simulink model "StopwatchAra2016"  (R2017b)
settings: Solver=ode3  StartTime=0.0  StopTime=Inf  RelTol=1e-3
libraries: simulink x1
settings Model: Creator=Gabriele Ara  LastModifiedBy=gabriele
settings OptimizationCC: DefaultParameterBehavior=Inlined  InlineInvariantSignals=on
settings DebuggingCC: ParameterTunabilityLossMsg=error
settings SFSimCC: MATLABDynamicMemAlloc=off
settings RTWCC: SystemTargetFile=ert.tlc  GenCodeOnly=on  TemplateMakefile=ert_default_tmf  GenerateReport=on  IncludeHyperlinkInReport=on  LaunchReport=on  GenerateTraceInfo=on  GenerateTraceReport=on  GenerateTraceReportSl=on  GenerateTraceReportSf=on  GenerateTraceReportEml=on
settings CodeAppCC: ForceParamTrailComments=on  IgnoreCustomStorageClasses=off  OperatorAnnotations=on  SimulinkDataObjDesc=on  SFDataObjDesc=on  MATLABFcnDesc=on  InsertBlockDesc=on  StateflowObjectComments=on  MATLABSourceComments=on
settings ERTTargetCC: TargetLangStandard=C99 (ISO)  MultiwordLength=2048  GenerateSampleERTMain=on  SupportAbsoluteTime=off  MultiInstanceERTCode=on  CodeInterfacePackaging=Reusable function  SupportNonFinite=off  SupportComplex=off  PurelyIntegerCode=on  InlinedParameterPlacement=NonHierarchical  MultiInstanceErrorCode=None  ERTCustomFileTemplate=example_file_process.tlc

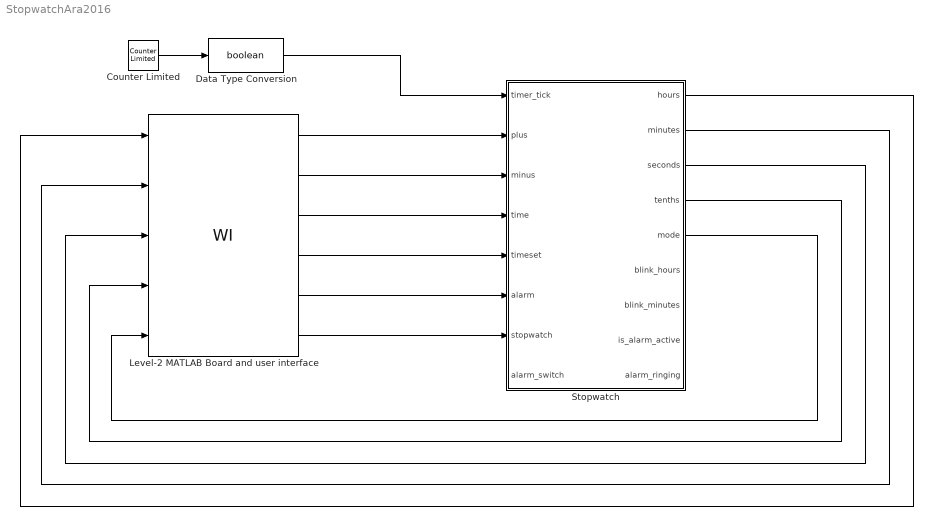
== system StopwatchAra2016 ==
  Counter Limited : simulink/Sources/Counter Limited  uplimit=1  tsamp=0.1
  Data Type Conversion : DataTypeConversion  OutDataTypeStr=boolean
  Level-2 MATLAB Board and user interface : M-S-Function  FunctionName=WI
      mask Display:
      | port_label('input', 1, 'hours')
      | port_label('input', 2, 'minutes')
      | port_label('input', 3, 'seconds')
      | port_label('input', 4, 'tenths')
      | port_label('input', 5, 'mode')
      | 
      | port_label('output', 1, 'plus')
      | port_label('output', 2, 'minus')
      | port_label('output', 3, 'time')
      | port_label('output', 4, 'time_set')
      | port_label('output', 5, 'alarm')
      | port_label('output', 6, 'stopwatch')
  Stopwatch : Subsystem
  wires:
  Level-2 MATLAB Board and user interface/1 -> Stopwatch/2(plus)
  Level-2 MATLAB Board and user interface/2 -> Stopwatch/3(minus)
  Level-2 MATLAB Board and user interface/3 -> Stopwatch/4(time)
  Level-2 MATLAB Board and user interface/4 -> Stopwatch/5(timeset)
  Level-2 MATLAB Board and user interface/5 -> Stopwatch/6(alarm)
  Level-2 MATLAB Board and user interface/6 -> Stopwatch/7(stopwatch)
  Stopwatch/1(hours) -> Level-2 MATLAB Board and user interface/1
  Stopwatch/2(minutes) -> Level-2 MATLAB Board and user interface/2
  Stopwatch/3(seconds) -> Level-2 MATLAB Board and user interface/3
  Stopwatch/4(tenths) -> Level-2 MATLAB Board and user interface/4
  Stopwatch/5(mode) -> Level-2 MATLAB Board and user interface/5
  Data Type Conversion/1 -> Stopwatch/1(timer_tick)
  Counter Limited/1 -> Data Type Conversion/1

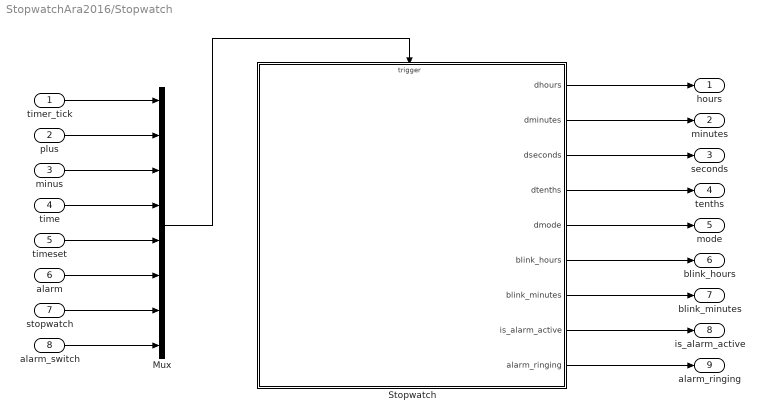
== system StopwatchAra2016/Stopwatch ==
  timer_tick : Inport
  plus : Inport  Port=2
  minus : Inport  Port=3
  time : Inport  Port=4
  timeset : Inport  Port=5
  alarm : Inport  Port=6
  stopwatch : Inport  Port=7
  alarm_switch : Inport  Port=8
  Mux : Mux  Inputs=8
  Stopwatch : Stateflow chart  TreatAsAtomicUnit=on
  hours : Outport
  minutes : Outport  Port=2
  seconds : Outport  Port=3
  tenths : Outport  Port=4
  mode : Outport  Port=5
  blink_hours : Outport  Port=6
  blink_minutes : Outport  Port=7
  is_alarm_active : Outport  Port=8
  alarm_ringing : Outport  Port=9
  wires:
  plus/1 -> Mux/2
  Stopwatch/1(dhours) -> hours/1
  minus/1 -> Mux/3
  timeset/1 -> Mux/5
  alarm/1 -> Mux/6
  time/1 -> Mux/4
  stopwatch/1 -> Mux/7
  Stopwatch/2(dminutes) -> minutes/1
  Stopwatch/5(dmode) -> mode/1
  Stopwatch/4(dtenths) -> tenths/1
  Stopwatch/3(dseconds) -> seconds/1
  Mux/1 -> Stopwatch/Trigger
  Stopwatch/8(is_alarm_active) -> is_alarm_active/1
  Stopwatch/7(blink_minutes) -> blink_minutes/1
  Stopwatch/6(blink_hours) -> blink_hours/1
  Stopwatch/9(alarm_ringing) -> alarm_ringing/1
  alarm_switch/1 -> Mux/8
  timer_tick/1 -> Mux/1

== stateflow chart StopwatchAra2016/Stopwatch/Stopwatch ==
  settings: executeAtInitialization=1
  state Control [parallel]
    en: blink_hours = uint8(0); blink_minutes = uint8(0);
    settings: executionOrder=1
    state timemode
      en: dmode = uint8(0);
      du: dhours = hours; dminutes = minutes; dseconds = seconds; dtenths = tenths;
    state timesetmode
      en: dmode = uint8(1); dhours = hours; dminutes = minutes;
      ex: hours = dhours; minutes = dminutes;
      state setMinutes
        en: blink_minutes = uint8(1);
        ex: blink_minutes = uint8(0);
        setMinutes -> setMinutes [order 1] : bplus {dminutes = mod(dminutes + 1, 60)}
        setMinutes -> setMinutes [order 2] : bminus [dminutes == 0]{dminutes = uint8(59)}
        setMinutes -> setMinutes [order 3] : bminus {dminutes = dminutes - 1}
      state setHours
        en: blink_hours = uint8(1);
        ex: blink_hours = uint8(0);
        setHours -> setHours [order 1] : bplus {dhours = mod(dhours + 1, 24)}
        setHours -> setHours [order 2] : bminus [dhours == 0]{dhours = uint8(23)}
        setHours -> setHours [order 3] : bminus {dhours = dhours - 1}
      (default) -> setHours
      setHours -> setMinutes [order 1] : timeset
      setMinutes -> setHours [order 1] : timeset
    state alarmmode
      en: dmode = uint8(2); dhours = alarm_hours; dminutes = alarm_minutes;
      du: dhours = alarm_hours; dminutes = alarm_minutes;
      state setAlarmHours
        en: blink_hours = uint8(1);
        ex: blink_hours = uint8(0);
        setAlarmHours -> setAlarmHours [order 1] : bplus {alarm_hours = mod(alarm_hours + 1, 24)}
        setAlarmHours -> setAlarmHours [order 2] : bminus [alarm_hours == 0]{alarm_hours = uint8(23)}
        setAlarmHours -> setAlarmHours [order 3] : bminus {alarm_hours = alarm_hours - 1}
      state setAlarmMinutes
        en: blink_minutes = uint8(1);
        ex: blink_minutes = uint8(0);
        setAlarmMinutes -> setAlarmMinutes [order 1] : bplus {alarm_minutes = mod(alarm_minutes + 1, 60)}
        setAlarmMinutes -> setAlarmMinutes [order 2] : bminus [alarm_minutes == 0]{alarm_minutes = uint8(59)}
        setAlarmMinutes -> setAlarmMinutes [order 3] : bminus {alarm_minutes = alarm_minutes - 1}
      (default) -> setAlarmHours
      setAlarmHours -> setAlarmMinutes [order 1] : alarm
      setAlarmMinutes -> setAlarmHours [order 1] : alarm
    state stopwatchmode
      en: dmode = uint8(3);
      state stopwatchOff
        en: s_hours = uint8(0); s_minutes = uint8(0); s_seconds = uint8(0); s_tenths = uint8(0); dtenths = s_tenths; dseconds = s_seconds; dminutes = s_minutes; dhours = s_hours;
      state stopwatchRunning
        en: s_running = uint8(1);
        ex: s_running = uint8(0);
        state running
          du: dtenths = s_tenths; dseconds = s_seconds; dminutes = s_minutes; dhours = s_hours;
        state showLap
        (default) -> running
        running -> showLap : bminus
        showLap -> running : bminus
      state stopwatchPaused
        en: dtenths = s_tenths; dseconds = s_seconds; dminutes = s_minutes; dhours = s_hours;
      (default) -> stopwatchOff
      stopwatchmode -> stopwatchOff [order 1] : stopwatch
      stopwatchOff -> stopwatchRunning : bplus
      stopwatchRunning -> stopwatchPaused : bplus
      stopwatchPaused -> stopwatchRunning : bplus
    timemode -> stopwatchmode [order 2] : stopwatch
    (default) -> timemode
    timemode -> timesetmode [order 1] : timeset
    Control -> timemode : time
    timesetmode -> alarmmode [order 1] : alarm
    timemode -> alarmmode [order 3] : alarm
    alarmmode -> timesetmode [order 1] : timeset
    stopwatchmode -> timesetmode [order 1] : timeset
    timesetmode -> stopwatchmode [order 2] : stopwatch
    stopwatchmode -> alarmmode [order 2] : alarm
    alarmmode -> stopwatchmode [order 2] : stopwatch
  state Timecount [parallel]
    en: hours = uint8(0); minutes = uint8(0); seconds = uint8(0); tenths = uint8(0); s_hours = uint8(0); s_minutes = uint8(0); s_seconds = uint8(0); s_tenths = uint8(0); s_running = uint8(0);
    settings: executionOrder=2
    (junction 174) -> (junction 199) [order 1] : [s_running == 1]
    Timecount -> (junction 174) : timer_tick
    (junction 174) -> (junction 176) [order 2]
    (junction 199) -> (junction 206) : {s_tenths = mod(s_tenths+1, 10)}
    (junction 210) -> (junction 176)
    (junction 206) -> (junction 210) [order 2]
    (junction 211) -> (junction 210)
    (junction 206) -> (junction 200) [order 1] : [s_tenths == 0] {s_seconds = mod(s_seconds+1, 60)}
    (junction 176) -> (junction 63) : {tenths = mod(tenths+1, 10)}
    (junction 63) -> Timecount [order 2]
    (junction 200) -> (junction 211) [order 2]
    (junction 63) -> (junction 64) [order 1] : [tenths == 0] {seconds = mod(seconds+1, 60)}
    (junction 200) -> (junction 203) [order 1] : [s_seconds == 0] {s_minutes = mod(s_minutes+1, 60)}
    (junction 212) -> (junction 211)
    (junction 64) -> Timecount [order 2]
    (junction 203) -> (junction 212) [order 2]
    (junction 64) -> (junction 65) [order 1] : [seconds == 0] {minutes = mod(minutes+1, 60)}
    (junction 201) -> (junction 212)
    (junction 203) -> (junction 201) [order 1] : [s_minutes == 0] {s_hours = mod(s_hours+1, 24)}
    (junction 65) -> Timecount [order 2]
    (junction 65) -> (junction 66) [order 1] : [minutes == 0] {hours = mod(hours+1, 24)}
    (junction 66) -> Timecount
  state Alarmmanage [parallel]
    en: alarm_hours = uint8(0); alarm_minutes = uint8(0); is_alarm_active = uint8(0); alarm_ringing = uint8(0);
    settings: executionOrder=3
    state alarmOff
      en: is_alarm_active = uint8(0);
    state alarmOn
      en: is_alarm_active = uint8(1);
      state waiting_next_activation
      state ringing
        en: alarm_ringing = uint8(1);
        ex: alarm_ringing = uint8(0);
      state quiet
      waiting_next_activation -> quiet : timer_tick [alarm_hours ~= hours && alarm_minutes ~= minutes]
      ringing -> waiting_next_activation [order 1] : alarm
      quiet -> ringing : timer_tick [alarm_hours == hours && alarm_minutes == minutes]
      ringing -> quiet [order 2] : timer_tick [alarm_hours ~= hours && alarm_minutes ~= minutes]
      (junction 232) -> quiet [order 2]
      (junction 232) -> ringing [order 1] : [alarm_hours == hours && alarm_minutes == minutes]
      (default) -> (junction 232)
    (default) -> alarmOff
    alarmOff -> alarmOn : alarm_switch
    alarmOn -> alarmOff : alarm_switch
  data: dhours output uint8; dminutes output uint8; dseconds output uint8; dtenths output uint8; dmode output uint8; hours local uint8; minutes local uint8; seconds local uint8; tenths local uint8; alarm_hours local uint8; alarm_minutes local uint8; blink_hours output uint8; blink_minutes output uint8; is_alarm_active output uint8; alarm_ringing output uint8; s_tenths local uint8; s_seconds local uint8; s_minutes local uint8; s_hours local uint8; s_running local uint8
  events: timer_tick input EITHER_EDGE_EVENT; bplus input RISING_EDGE_EVENT; bminus input RISING_EDGE_EVENT; time input RISING_EDGE_EVENT; timeset input RISING_EDGE_EVENT; alarm input RISING_EDGE_EVENT; stopwatch input RISING_EDGE_EVENT; alarm_switch input RISING_EDGE_EVENT
